simulink model "s1"  (Simulink 2.00)
settings: Solver=ode15s  StartTime=0.0  StopTime=2  MaxStep=1e-3  RelTol=1e-6  AbsTol=1e-6
values from neighbouring files (symbols this model uses):
  Ia = [ -40:5:40]    [M1.M]
  Iar = 0.04*abs(atan(Ia)) + 0.0001*Ia.^2    [M1.M]
  Laq = 0.018    [M1.M]    (also in M2.M = 0.012; M3A.M; M3B.M; M4.M = 0.01)
  Lf = 10    [M1.M]    (also in M3A.M; M3B.M)
  Ra = 0.24    [M1.M]    (also in M2.M = 0.3; M3A.M = 0.14; M3B.M = 0.14; M4.M = 0.6)
  Rf = 111    [M1.M]    (also in M3A.M; M3B.M)
  Rload = 1e6    (= 1000000)    [M1.M]    (also in M3A.M)
  Rrh = 25    [M1.M]    (also in M3A.M; M3B.M)
  SHIP1 = [0 0.05 0.1 0.13 0.18 0.22 0.26 0.32 0.36 0.4 0.47 0.54   0.575 0.61 0.64 0.68 0.71 0.74 0.78 0.82 0.86 0.9 0.93 1.0 1.1   1.2 1.3 1.4 1.5]    [M1.M]
  SHVP1 = [7.5 12 20 24 32 40 48 59 66 74 86 97 102.5  107.5 112 117 121 125 130 135 140 143 146 152 158 164 168 172 175]    [M1.M]
  wmo = 2000*(2*pi)/60    (= 209.439510239)    [M1.M]    (also in M4.M = 157.079632679; M5.M = 125.663706144)
  wmrated = 1750*(2*pi)/60    (= 183.259571459)    [M1.M]    (also in M2.M = 156.032435128; M3A.M; M3B.M; M4.M = 293.215314335)
settings Model: SaveTime=off  SaveOutput=off  ConsistencyChecking=off

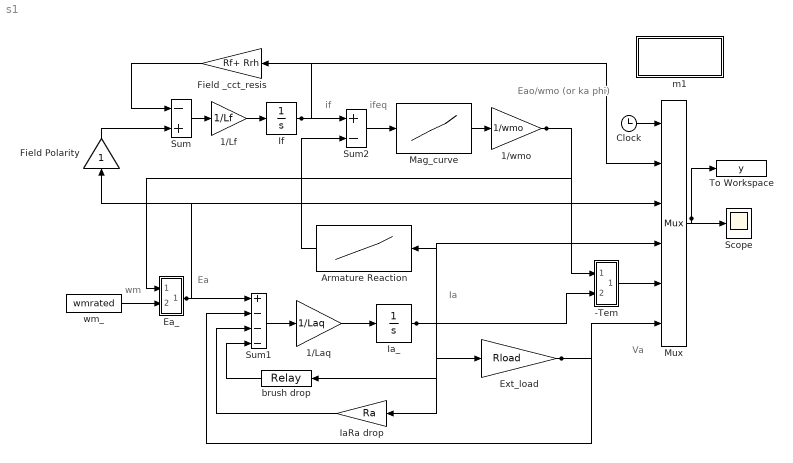
== system s1 ==
  note: if
  note: Eao/wmo
      | (or ka phi)
  note: wm
  note: Ea
  note: Ia
  note: ifeq
  note: Va
  -Tem : Subsystem
      mask Type: Dot Product
      mask Description:
      | Inner (dot) product.
      | y=sum(u1.*u2)
      mask Help: Computes the inner (dot) product of the inputs: sum(u1.*u2).  The inputs are vectors of the same length. Output is a scalar.
      mask Display: disp('.\n')
  1/Laq : Gain  Gain=1/Laq
  1/Lf : Gain  Gain=1/Lf
  1/wmo : Gain  Gain=1/wmo
  Armature Reaction : Lookup  Orientation=left  InputValues=Ia  OutputValues=Iar
  Clock : Clock
      settings: DeleteFcn=simclock BlockIsBeingDestroyed  PostSaveFcn=simclock Save
  Ea_ : Subsystem
      mask Type: Dot Product
      mask Description:
      | Inner (dot) product.
      | y=sum(u1.*u2)
      mask Help: Computes the inner (dot) product of the inputs: sum(u1.*u2).  The inputs are vectors of the same length. Output is a scalar.
      mask Display: disp('.\n')
  Ext_load : Gain  Gain=Rload
  Field Polarity : Gain  Orientation=up  Gain=1
  Field _cct_resis : Gain  Orientation=left  Gain=Rf+ Rrh
  IaRa drop : Gain  Orientation=left  Gain=Ra
  Ia_ : Integrator  ExternalReset=none  InitialConditionSource=internal  InitialCondition=0  LimitOutput=off  UpperSaturationLimit=inf  LowerSaturationLimit=-inf  ShowSaturationPort=off  ShowStatePort=off  AbsoluteTolerance=auto
  If : Integrator  ExternalReset=none  InitialConditionSource=internal  InitialCondition=0  LimitOutput=off  UpperSaturationLimit=inf  LowerSaturationLimit=-inf  ShowSaturationPort=off  ShowStatePort=off  AbsoluteTolerance=auto
  m1 : Subsystem
      settings: OpenFcn=m1
      mask Type: Masked block of m1.m
      mask Help: Uses m1.m to initialize and plot
      mask Display: disp('Initialize\nand plot')
  Mag_curve : Lookup  InputValues=SHIP1  OutputValues=SHVP1
  Mux : Mux  Inputs=6
  Scope : Scope
      settings: TickLabels=on  TimeRange=2.000000  YMin=-150.000000  YMax=150.000000  SaveToWorkspace=off  SaveName=ScopeData
  Sum : Sum  Inputs=-+
  Sum1 : Sum  Inputs=+---
  Sum2 : Sum  Inputs=+-
  To Workspace : ToWorkspace  VariableName=y  SampleTime=0
      settings: Buffer=5000
  brush drop : Relay  Orientation=left  OnSwitchValue=eps  OffSwitchValue=eps  OnOutputValue=2  OffOutputValue=-2
  wm_ : Constant  Value=wmrated
  wires:
  Sum/1 -> 1/Lf/1
  1/Lf/1 -> If/1
  Mag_curve/1 -> 1/wmo/1
  Sum1/1 -> 1/Laq/1
  1/Laq/1 -> Ia_/1
  Clock/1 -> Mux/1
  -Tem/1(out_1) -> Mux/5
  wm_/1 -> Ea_/2(in_2)
  Field _cct_resis/1 -> Sum/1
  Field Polarity/1 -> Sum/2
  Ia_/1 -> IaRa drop/1, -Tem/2(in_2), Armature Reaction/1, Mux/4, brush drop/1, Ext_load/1
  1/wmo/1 -> Ea_/1(in_1), -Tem/1(in_1)
  Ea_/1(out_1) -> Field Polarity/1, Mux/3, Sum1/1
  Sum2/1 -> Mag_curve/1
  Armature Reaction/1 -> Sum2/2
  If/1 -> Sum2/1, Field _cct_resis/1, Mux/2
  brush drop/1 -> Sum1/4
  IaRa drop/1 -> Sum1/3
  Ext_load/1 -> Mux/6, Sum1/2
  Mux/1 -> Scope/1, To Workspace/1

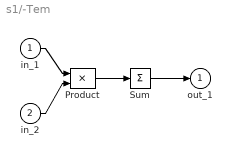
== system s1/-Tem ==
  in_1 : Inport  Port=1  PortWidth=-1  SampleTime=-1
  in_2 : Inport  Port=2  PortWidth=-1  SampleTime=-1
  Product : Product  Inputs=2
  Sum : Sum  Inputs=+
  out_1 : Outport  Port=1  InitialOutput=0
  wires:
  in_2/1 -> Product/2
  in_1/1 -> Product/1
  Product/1 -> Sum/1
  Sum/1 -> out_1/1

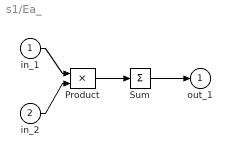
== system s1/Ea_ ==
  in_1 : Inport  Port=1  PortWidth=-1  SampleTime=-1
  in_2 : Inport  Port=2  PortWidth=-1  SampleTime=-1
  Product : Product  Inputs=2
  Sum : Sum  Inputs=+
  out_1 : Outport  Port=1  InitialOutput=0
  wires:
  in_2/1 -> Product/2
  in_1/1 -> Product/1
  Product/1 -> Sum/1
  Sum/1 -> out_1/1

== system s1/m1 ==
  note: Masked block of m1.m in Chapter 8
      | to initialize s1.m and plot results
